simulink model "t1q6"  (R2017b)
settings: Solver=VariableStepAuto  StartTime=0.0  StopTime=500  RelTol=1e-3
values from neighbouring files (symbols this model uses):
  Ca_0 = 0.7192    [t1.m]    (also in t1q5.m = double(max(solve(0 == -k1*Ca - k3*Ca^2 + (Caf_0 - Ca)*u_0,Ca; t1q9.m = double(max(solve(0 == -k1*Ca - k3*Ca^2 + (Caf_0 - Ca)*u_0,Ca)
  Cb_0 = 2.345    [t1.m]    (also in t1q5.m = double(solve(0 == k1*Ca_0 - k2*Cb - Cb*u_0, Cb)); t1q9.m = double(solve(0 == k1*Ca_0 - k2*Cb - Cb*u_0, Cb)))
  k1 = 6.01    [t1.m]    (also in t1q5.m; t1q9.m)
  k2 = 0.8433    [t1.m]    (also in t1q5.m; t1q9.m)
  k3 = 0.1123    [t1.m]    (also in t1q5.m; t1q9.m)
libraries: cstblocks x8
settings Model: Creator=vinic  LastModifiedBy=vinic

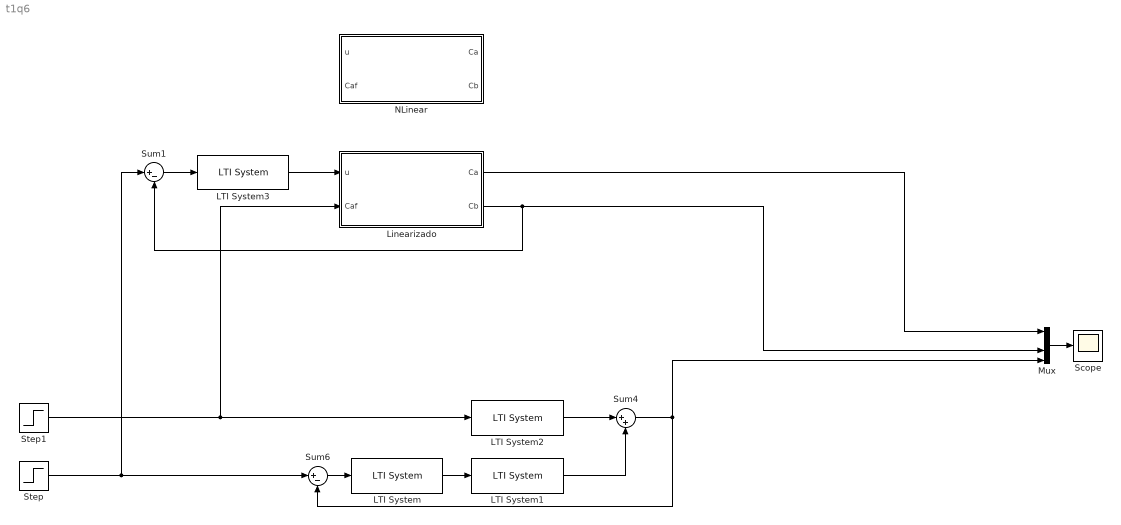
== system t1q6 ==
  LTI System : cstblocks/LTI System  sys=C  IC=[]
  LTI System1 : cstblocks/LTI System  sys=P  IC=[]
  LTI System2 : cstblocks/LTI System  sys=Q  IC=[]
  LTI System3 : cstblocks/LTI System  sys=C  IC=[]
  Linearizado : Subsystem
  Mux : Mux
  NLinear : Subsystem
  Scope : Scope
  Step : Step  Time=100  SampleTime=0
  Step1 : Step  Time=250  SampleTime=0
  Sum1 : Sum  Inputs=|+-
  Sum4 : Sum  Inputs=|++
  Sum6 : Sum  Inputs=|+-
  wires:
  Mux/1 -> Scope/1
  LTI System2/1 -> Sum4/1
  LTI System1/1 -> Sum4/2
  Sum4/1 -> Mux/4, Sum6/2
  LTI System/1 -> LTI System1/1
  Sum6/1 -> LTI System/1
  Step/1 -> Sum1/1, Sum6/1
  LTI System3/1 -> Linearizado/1(u)
  Sum1/1 -> LTI System3/1
  Linearizado/2(Cb) -> Sum1/2, Mux/3
  Step1/1 -> Linearizado/2(Caf), LTI System2/1
  Linearizado/1(Ca) -> Mux/1

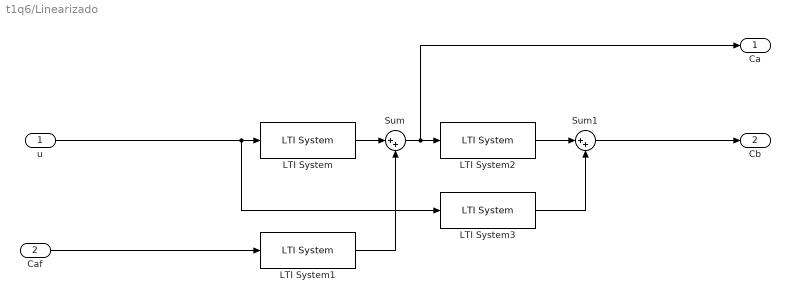
== system t1q6/Linearizado ==
  u : Inport
  Caf : Inport  Port=2
  LTI System : cstblocks/LTI System  sys=Ca_U  IC=[]
  LTI System1 : cstblocks/LTI System  sys=Ca_Caf  IC=[]
  LTI System2 : cstblocks/LTI System  sys=Cb_Ca  IC=[]
  LTI System3 : cstblocks/LTI System  sys=Cb_U  IC=[]
  Sum : Sum  Inputs=|++
  Sum1 : Sum  Inputs=|++
  Ca : Outport
  Cb : Outport  Port=2
  wires:
  u/1 -> LTI System3/1, LTI System/1
  Caf/1 -> LTI System1/1
  LTI System1/1 -> Sum/2
  LTI System/1 -> Sum/1
  Sum/1 -> Ca/1, LTI System2/1
  Sum1/1 -> Cb/1
  LTI System2/1 -> Sum1/1
  LTI System3/1 -> Sum1/2

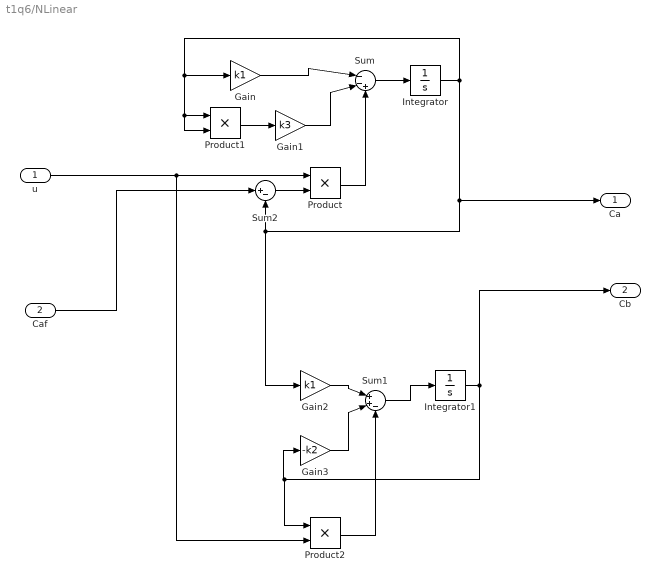
== system t1q6/NLinear ==
  u : Inport
  Caf : Inport  Port=2
  Gain : Gain  Gain=k1
  Gain1 : Gain  Gain=k3
  Gain2 : Gain  Gain=k1
  Gain3 : Gain  Gain=-k2
  Integrator : Integrator  InitialCondition=Ca_0
  Integrator1 : Integrator  InitialCondition=Cb_0
  Product : Product
  Product1 : Product
  Product2 : Product
  Sum : Sum  Inputs=|--+
  Sum1 : Sum  Inputs=|++-
  Sum2 : Sum  Inputs=|+-
  Ca : Outport
  Cb : Outport  Port=2
  wires:
  Sum/1 -> Integrator/1
  Integrator1/1 -> Cb/1, Product2/1, Gain3/1
  Caf/1 -> Sum2/1
  u/1 -> Product2/2, Product/1
  Integrator/1 -> Ca/1, Gain2/1, Sum2/2, Product1/1, Product1/2, Gain/1
  Sum2/1 -> Product/2
  Gain/1 -> Sum/1
  Product/1 -> Sum/3
  Gain3/1 -> Sum1/2
  Product2/1 -> Sum1/3
  Sum1/1 -> Integrator1/1
  Gain1/1 -> Sum/2
  Product1/1 -> Gain1/1
  Gain2/1 -> Sum1/1
